simulink model "KAL_MPC"  (R2019a)
settings: Solver=FixedStepAuto  StartTime=0.0  StopTime=4/speed  FixedStep=0.005  MaxStep=1e-2  MinStep=1e-3  RelTol=5e-3
PreLoadFcn:
  | helperSLCreateUtilityBus;
  | createCostmap;
StopFcn:
  | clear helperSLVisualizePath;
values from neighbouring files (symbols this model uses):
  costmap = vehicleCostmap(circuit, 'cellSize', res )    [createCostmap.m]    (also in helperSLVisualizePath.m = vehicleCostmap(costmapStruct.Costs,          'FreeThreshold')
  curvatures = zeros(561,1)    [createCostmap.m]
  directions = ones(561,1)    [createCostmap.m]
  refPoses = zeros(561, 3)    [createCostmap.m]
  speed = 0.1    [createCostmap.m]
  speedprofile = ones(561,1).*speed    [createCostmap.m]
  startPose = refPoses(1,:)    [createCostmap.m]
  wheelbase = 0.3    [createCostmap.m]
libraries: simulink_extras x2, autolibshared x1
settings Model: Creator=The MathWorks, Inc.  LastModifiedBy=mingz
settings SolverCC: ZeroCrossAlgorithm=Adaptive  DecoupledContinuousIntegration=on  MinimalZcImpactIntegration=on
settings DataIOCC: SaveOutput=off  SignalLogging=off  DSMLogging=off  SaveTime=off  ReturnWorkspaceOutputs=off
settings DebuggingCC: PregeneratedLibrarySubsystemCodeDiagnostic=none  ArithmeticOperatorsInVariantConditions=warning
settings SFSimCC: SimUseLocalCustomCode=off
settings RTWCC: RTWUseLocalCustomCode=off

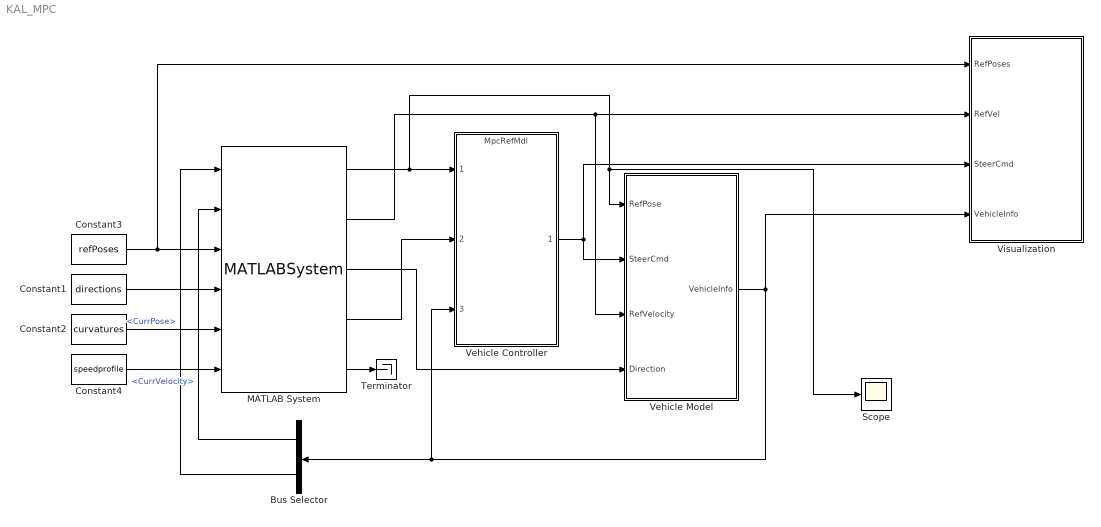
== system KAL_MPC ==
  Bus Selector : BusSelector  OutputSignals=CurrVelocity,CurrPose
  Constant1 : Constant  Value=directions
  Constant2 : Constant  Value=curvatures
  Constant3 : Constant  Value=refPoses
  Constant4 : Constant  Value=speedprofile
  MATLAB System : MATLABSystem  System=HelperPathAnalyzer  Wheelbase=wheelbase  HasResetOutput=on  SimulateUsing=Interpreted execution
      mask Type: HelperPathAnalyzer
      mask Display:
      | disp(['Helper' char(10) 'Path' char(10) 'Analyzer']);
      | port_label('input',1,'CurrPose');
      | port_label('input',2,'CurrVelocity');
      | port_label('input',3,'RefPoses');
      | port_label('input',4,'Directions');
      | port_label('input',5,'Curvatures');
      | port_label('input',6,'SpeedProfile');
      | port_label('output',1,'RefPose');
      | port_label('output',2,'RefVelocity');
      | port_label('output',3,'Direction');
      | port_label('output',4,'Curvature');
      | port_label('output',5,'Reset');
  Scope : Scope
  Terminator : Terminator
  Vehicle Controller : ModelReference  ModelNameDialog=MpcRefMdl.slx  SimulationMode=Normal  ModelReferenceVersion=1.1095
  Vehicle Model : Subsystem
  Visualization : Subsystem  mask{Costmap=costmap}
      mask prompts: Costmap "Vehicle costmap:"
      mask init:
      | validateattributes(Costmap, {'vehicleCostmap'}, {'scalar'});
      | 
      | varagout          = helperSLCreateUtilityStruct(Costmap);
      | vehicleDimsStruct = varagout{1};
      | costmapStruct     = varagout{2};
      mask DialogControl DescTextVar Prompt: Visualize simulation results.
  wires:
  Bus Selector/2 -> MATLAB System/1  "<CurrPose>"
  Bus Selector/1 -> MATLAB System/2  "<CurrVelocity>"
  MATLAB System/4 -> Vehicle Controller/2
  Vehicle Model/1(VehicleInfo) -> Visualization/4(VehicleInfo), Vehicle Controller/3, Bus Selector/1
  Constant1/1 -> MATLAB System/4
  Constant2/1 -> MATLAB System/5
  Constant4/1 -> MATLAB System/6
  Constant3/1 -> Visualization/1(RefPoses), MATLAB System/3
  MATLAB System/1 -> Vehicle Model/1(RefPose), Scope/1, Vehicle Controller/1
  MATLAB System/2 -> Vehicle Model/3(RefVelocity), Visualization/2(RefVel)
  Vehicle Controller/1 -> Vehicle Model/2(SteerCmd), Visualization/3(SteerCmd)
  MATLAB System/5 -> Terminator/1
  MATLAB System/3 -> Vehicle Model/4(Direction)

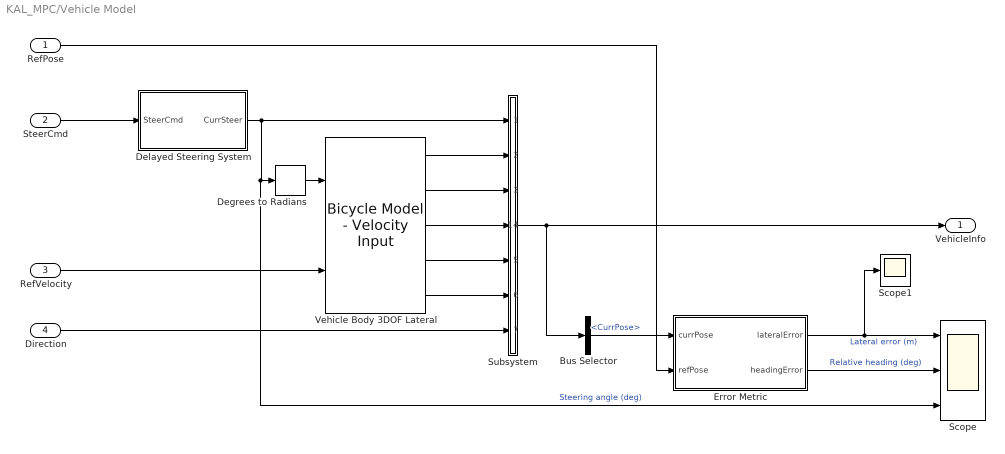
== system KAL_MPC/Vehicle Model ==
  RefPose : Inport
  SteerCmd : Inport  Port=2
  RefVelocity : Inport  Port=3
  Direction : Inport  Port=4
  Bus Selector : BusSelector  OutputSignals=CurrPose
  Degrees to Radians : simulink_extras/Transformations/Degrees to Radians
  Delayed Steering System : Subsystem
  Error Metric : MATLAB Function  TreatAsAtomicUnit=on  mask{wheelbase=wheelbase}
      mask prompts: wheelbase "Wheelbase of vehicle"
  Scope : Scope  NumInputPorts=3
  Scope1 : Scope
  Subsystem : Subsystem
  Vehicle Body 3DOF Lateral : autolibshared/Bicycle Model - Velocity Input  trackMode=Single (bicycle)  inputMode=External longitudinal forces  frontSteerMode=on  rearSteerMode=off  windMode=off  muMode=off  extFMode=off  extMMode=off  aMode=3  NF=2  NR=2  m=1.2  a=0.10  b=0.05  h=0.04  X_o=startPose(1)+cosd(startPose(3))*0.05  xdot_o=0  CalphaMode=off  sigmaMode=on  w=[1.4,1.4]  Cy_f=19e3  Cy_r=20e3  sigma_f=.1  sigma_r=.1  alpha_f_brk=[-.1 .1]  Cy_f_data=[-9e3 9e3]  alpha_r_brk=[-.1 .1]  Cy_r_data=[-9e3 9e3]  Y_o=startPose(2)+sind(startPose(3))*0.05  ydot_o=0  Izz=0.004  psi_o=deg2rad(startPose(3))  r_o=0  Af=2  Cd=.3  Cl=.1  Cpm=.1  beta_w=[0:0.01:0.3]  Cs=[0:0.03:0.9]  Cym=[0:0.01:0.3]  Pabs=101325  Tair=273  g=9.81  mu=1  xdot_tol=0.01  Fznom=5000  Fxtire_sat=1e6  Fytire_sat=1e6  longOff=0  latOff=0  vertOff=0
      settings: SourceProductName=Powertrain Blockset  SourceProductBaseCode=PW
  VehicleInfo : Outport
  wires:
  RefVelocity/1 -> Vehicle Body 3DOF Lateral/2
  Direction/1 -> Subsystem/7(<Direction>)
  Degrees to Radians/1 -> Vehicle Body 3DOF Lateral/1
  SteerCmd/1 -> Delayed Steering System/1(SteerCmd)
  Subsystem/1(VehicleInfo) -> Bus Selector/1, VehicleInfo/1
  Vehicle Body 3DOF Lateral/1 -> Subsystem/2(Info)
  Vehicle Body 3DOF Lateral/2 -> Subsystem/3(In3)
  Vehicle Body 3DOF Lateral/3 -> Subsystem/4(In4)
  Vehicle Body 3DOF Lateral/4 -> Subsystem/5(In5)
  Vehicle Body 3DOF Lateral/5 -> Subsystem/6(In6)
  Error Metric/2(headingError) -> Scope/2  "Relative heading (deg)"
  Error Metric/1(lateralError) -> Scope1/1, Scope/1  "Lateral error (m)"
  Delayed Steering System/1(CurrSteer) -> Scope/3, Degrees to Radians/1, Subsystem/1(CurrSteer)  "Steering angle (deg)"
  RefPose/1 -> Error Metric/2(refPose)
  Bus Selector/1 -> Error Metric/1(currPose)  "<CurrPose>"

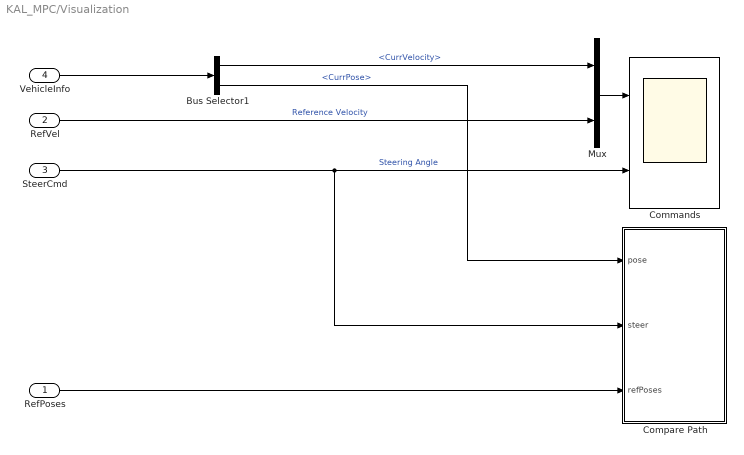
== system KAL_MPC/Visualization ==
  RefPoses : Inport
  RefVel : Inport  Port=2
  SteerCmd : Inport  Port=3
  VehicleInfo : Inport  Port=4
  Bus Selector1 : BusSelector  OutputSignals=CurrVelocity,CurrPose
  Commands : Scope  NumInputPorts=2
  Compare Path : MATLAB Function  TreatAsAtomicUnit=on
  Mux : Mux  Inputs=2
  wires:
  Bus Selector1/1 -> Mux/1  "<CurrVelocity>"
  Bus Selector1/2 -> Compare Path/1(pose)  "<CurrPose>"
  RefVel/1 -> Mux/2  "Reference Velocity"
  Mux/1 -> Commands/1
  SteerCmd/1 -> Compare Path/2(steer), Commands/2  "Steering Angle"
  VehicleInfo/1 -> Bus Selector1/1
  RefPoses/1 -> Compare Path/3(refPoses)

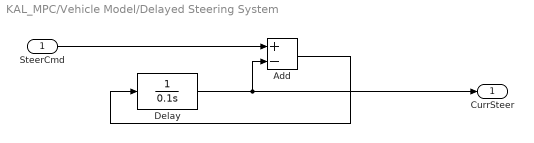
== system KAL_MPC/Vehicle Model/Delayed Steering System ==
  SteerCmd : Inport
  Add : Sum  Inputs=+-
  Delay : TransferFcn  Denominator=[0.1 0]
  CurrSteer : Outport
  wires:
  Add/1 -> Delay/1
  SteerCmd/1 -> Add/1
  Delay/1 -> CurrSteer/1, Add/2

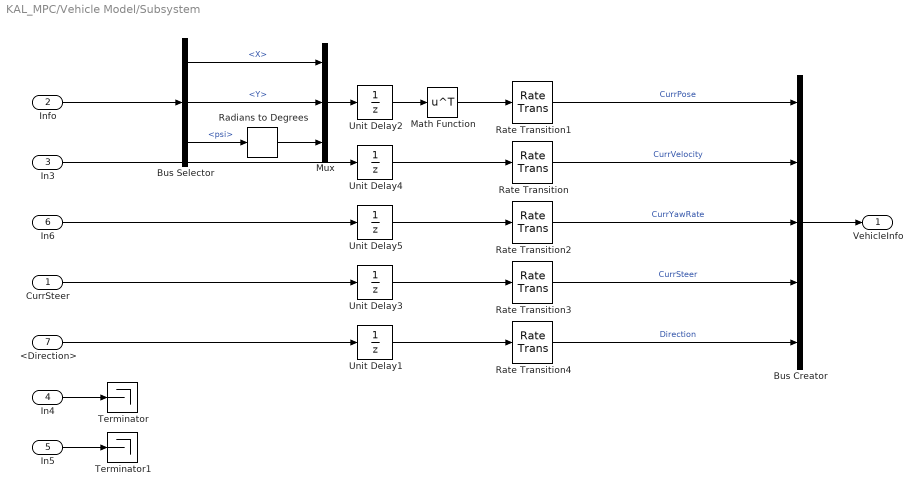
== system KAL_MPC/Vehicle Model/Subsystem ==
  CurrSteer : Inport
  Info : Inport  Port=2
  In3 : Inport  Port=3
  In4 : Inport  Port=4
  In5 : Inport  Port=5
  In6 : Inport  Port=6
  <Direction> : Inport  Port=7
  Bus Creator : BusCreator  Inputs=5  OutDataTypeStr=Bus: vehicleInfoBus  NonVirtualBus=on
  Bus Selector : BusSelector  OutputSignals=InertFrm.RearAxl.Disp.X,InertFrm.RearAxl.Disp.Y,InertFrm.Cg.Ang.psi
  Math Function : Math  Operator=transpose  SaturateOnIntegerOverflow=on
  Mux : Mux  Inputs=3
  Radians to Degrees : simulink_extras/Transformations/Radians to Degrees
  Rate Transition : RateTransition  InitialCondition=speed  OutPortSampleTime=0.005
  Rate Transition1 : RateTransition  InitialCondition=startPose  OutPortSampleTime=0.005
  Rate Transition2 : RateTransition  OutPortSampleTime=0.005
  Rate Transition3 : RateTransition  OutPortSampleTime=0.005
  Rate Transition4 : RateTransition  InitialCondition=1  OutPortSampleTime=0.005
  Terminator : Terminator
  Terminator1 : Terminator
  Unit Delay1 : UnitDelay  InitialCondition=1  SampleTime=-1  HasFrameUpgradeWarning=on
  Unit Delay2 : UnitDelay  InitialCondition=startPose  SampleTime=-1  HasFrameUpgradeWarning=on
  Unit Delay3 : UnitDelay  SampleTime=-1  HasFrameUpgradeWarning=on
  Unit Delay4 : UnitDelay  InitialCondition=speed  SampleTime=-1  HasFrameUpgradeWarning=on
  Unit Delay5 : UnitDelay  SampleTime=-1  HasFrameUpgradeWarning=on
  VehicleInfo : Outport
  wires:
  Unit Delay1/1 -> Rate Transition4/1
  CurrSteer/1 -> Unit Delay3/1
  Unit Delay5/1 -> Rate Transition2/1
  <Direction>/1 -> Unit Delay1/1
  Unit Delay4/1 -> Rate Transition/1
  Math Function/1 -> Rate Transition1/1
  Rate Transition/1 -> Bus Creator/2  "CurrVelocity"
  Unit Delay3/1 -> Rate Transition3/1
  Rate Transition3/1 -> Bus Creator/4  "CurrSteer"
  Rate Transition1/1 -> Bus Creator/1  "CurrPose"
  Rate Transition2/1 -> Bus Creator/3  "CurrYawRate"
  Rate Transition4/1 -> Bus Creator/5  "Direction"
  In5/1 -> Terminator1/1
  Unit Delay2/1 -> Math Function/1
  Info/1 -> Bus Selector/1
  Radians to Degrees/1 -> Mux/3
  Bus Selector/2 -> Mux/2  "<Y>"
  Bus Selector/1 -> Mux/1  "<X>"
  Mux/1 -> Unit Delay2/1
  In3/1 -> Unit Delay4/1
  In4/1 -> Terminator/1
  In6/1 -> Unit Delay5/1
  Bus Selector/3 -> Radians to Degrees/1  "<psi>"
  Bus Creator/1 -> VehicleInfo/1

== matlab function KAL_MPC/Vehicle Model/Error Metric ==
  data: currPose input size=[1 3]; refPose input size=[1 3]; lateralError output; wheelbase parameter; headingError output
function [lateralError, headingError] = fcn(currPose, refPose, wheelbase)

%   Copyright 2018 The MathWorks, Inc.

currPose(:,3) = deg2rad(currPose(:,3));
refPose(:,3)  = deg2rad(refPose(:,3));

%Convert current pose to front wheel coordinate
currPoseF = coder.nullcopy(zeros(1, 3));

currPoseF = driving.internal.control.rearPoseToFrontPose(currPose, wheelbase);

lateralError = norm(currPoseF(1:2) - refPose(1:2));

d1 = rad2deg(currPose(:, 3) - refPose(:,3));
d2 = 360 - abs(d1);
if (d1>0)
    d2 = 0.0-d2;
end
if (abs(d1) < abs(d2))
    headingError = d1;
else
    headingError = d2;
end

== matlab function KAL_MPC/Visualization/Compare Path ==
  settings: updateMethod=DISCRETE  sampleTime=0.1
  data: pose input size=[1 3]; steer input; refPoses input; costmapStruct parameter; vehicleDimsStruct parameter
function visualizePath(pose, steer, refPoses, costmapStruct, vehicleDimsStruct)

%visualizePath Display simulation results.

coder.extrinsic('helperSLVisualizePath');

helperSLVisualizePath(pose, steer, refPoses, costmapStruct, vehicleDimsStruct)
